simulink model "Switch_Block_1"  (R2021a)
settings: Solver=VariableStepAuto  StartTime=0.0  StopTime=10.0  MaxStep=1e-3  RelTol=1e-3
settings Model: Creator=lenovo  LastModifiedBy=lenovo

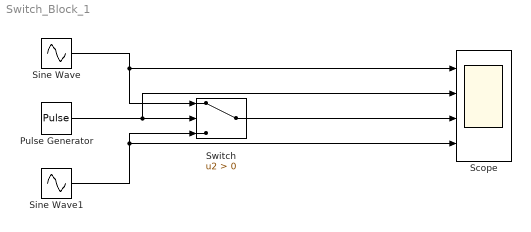
== system Switch_Block_1 ==
  Pulse Generator : DiscretePulseGenerator  PulseType=Time based  Period=1  PulseWidth=50
  Scope : Scope  NumInputPorts=4
  Sine Wave : Sin  SampleTime=0
  Sine Wave1 : Sin  Phase=-pi  SampleTime=0
  Switch : Switch  Criteria=u2 > Threshold
  wires:
  Pulse Generator/1 -> Scope/2, Switch/2
  Sine Wave1/1 -> Scope/4, Switch/3
  Sine Wave/1 -> Switch/1, Scope/1
  Switch/1 -> Scope/3
